simulink model "MotionControl"  (R2014a)
settings: Solver=ode45  StartTime=0.0  StopTime=40  FixedStep=0.00001  RelTol=1e-3
settings Model: Creator=faezeh  LastModifiedBy=faezeh

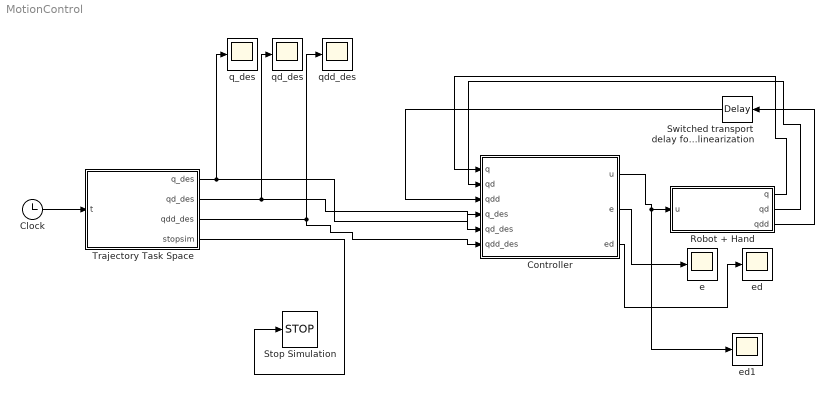
== system MotionControl ==
  Clock : Clock
  Controller : MATLAB Function  TreatAsAtomicUnit=on
  "Robot + Hand " : Subsystem
  Stop Simulation : Stop
  Switched transport delay for linearization : TransportDelay  DelayTime=0.001  TransDelayFeedthrough=on  PadeOrder=2
  Trajectory Task Space : MATLAB Function  TreatAsAtomicUnit=on
  e : Scope
      settings: YMin=-0.0025  YMax=0.0525  SaveName=ScopeData3
  ed : Scope
      settings: TimeRange=40  YMin=-0.05  YMax=1.1  SaveName=ScopeData4
  ed1 : Scope
      settings: YMin=0.00025  YMax=0.00425  SaveName=ScopeData5
  q_des : Scope
      settings: YMin=0.00025  YMax=0.00425
  qd_des : Scope
  qdd_des : Scope
      settings: SaveName=ScopeData2
  wires:
  Clock/1 -> Trajectory Task Space/1(t)
  Trajectory Task Space/1(q_des) -> q_des/1, Controller/4(q_des)
  Trajectory Task Space/2(qd_des) -> qd_des/1, Controller/5(qd_des)
  Trajectory Task Space/3(qdd_des) -> qdd_des/1, Controller/6(qdd_des)
  Controller/1(u) -> ed1/1, "Robot + Hand "/1("u ")
  Trajectory Task Space/4(stopsim) -> Stop Simulation/1
  "Robot + Hand "/1(q) -> Controller/1(q)
  "Robot + Hand "/2(qd) -> Controller/2(qd)
  Controller/2(e) -> e/1
  Controller/3(ed) -> ed/1
  "Robot + Hand "/3(qdd) -> Switched transport delay for linearization/1
  Switched transport delay for linearization/1 -> Controller/3(qdd)

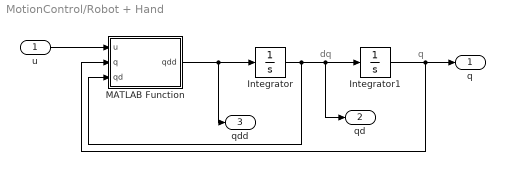
== system MotionControl/Robot + Hand  ==
  note: q
  note: dq
  "u " : Inport
  Integrator : Integrator  InitialCondition=[0.0;0.0;0.0]
  Integrator1 : Integrator  InitialCondition=[0.0;0.0;0.0]
  MATLAB Function : MATLAB Function  TreatAsAtomicUnit=on
  q : Outport
  qd : Outport  Port=2
  qdd : Outport  Port=3
  wires:
  "u "/1 -> MATLAB Function/1(u)
  Integrator/1 -> MATLAB Function/3(qd), qd/1, Integrator1/1
  Integrator1/1 -> MATLAB Function/2(q), q/1
  MATLAB Function/1(qdd) -> qdd/1, Integrator/1

== matlab function MotionControl/Robot + Hand /MATLAB Function ==
  data: u input; qdd output; q input; qd input
function qdd = DirDyn(u,q,qd)
%% Recalling Model Dynamics 
[M,V,G] = DynamicModel(q,qd);
B=[0.0252; 0.0019; 0.0029]; %Nms/rad
Fk=[0.1891; 0.0541; 0.1339]*0;
Jmeta=35.9*0.9*0.9*[1;1;1]*0.001*0.0001;
M=M+[Jmeta(1) 0 0;0 Jmeta(2) 0;0 0 Jmeta(3)]; 
%% Recalling Model Dynamics 
% [~,J,~] = DH2TF(q(1),q(2),q(3));
q1=q(1); q2=q(2); q3=q(3);
J=[ 0,        0,                       0
 0,        0,                       0
 0,        0,                       0
 0, -sin(q1), -cos(q1)*sin(q2 - pi/2)
 0,  cos(q1), -sin(q1)*sin(q2 - pi/2)
 1,        0,          cos(q2 - pi/2)];
fg = -4.98 + 16.92./((1+q./8.59).^2.24);
tawe = fg*66.457*0.001;
qdd =inv(M)*(u -(V + G + B.*qd + Fk.*sign(qd) + tawe));

== matlab function MotionControl/Controller ==
  data: q input; u output; qd input; qdd input; q_des input; qd_des input; qdd_des input; e output; ed output
function [u,e,ed] =Commanand (q,qd,qdd,q_des,qd_des,qdd_des)
    %% Recalling Model Dynamics 
    [M,V,G] = DynamicModel(q,qd);
    B=[0.0252; 0.0019; 0.0029]; %Nms/rad
    Fk=[0.1891; 0.0541; 0.1339]*0; %Nm
    Jmeta=35.9*0.9*0.9*[1;1;1]*0.001*0.0001;
    M=M+[Jmeta(1) 0 0;0 Jmeta(2) 0;0 0 Jmeta(3)];
%     qdd=[0;0;0];
    %% Recalling Model Kinematics
%     [~,J,~] = DH2TF(q(1),q(2),q(3));
    q1=q(1); q2=q(2); q3=q(3);
%     J=[ 0,        0,                    0
%      0,        0,                       0
%      0,        0,                       0
%      0, -sin(q1), -cos(q1)*sin(q2 - pi/2)
%      0,  cos(q1), -sin(q1)*sin(q2 - pi/2)
%      1,        0,          cos(q2 - pi/2)];
    %% Controller Command
    kp=4000;
    kd=1000;
%     q=[0;0;0];
%     qd=[0;0;0];   
u = M*(qdd_des+kd*(qd_des-qd)+kp*(q_des-q)) + V + G + B.*qd + Fk.*sign(qd);  
e=q_des-q;
    ed=qd_des-qd;

== matlab function MotionControl/Trajectory Task Space ==
  data: t input; q_des output; qd_des output; qdd_des output; stopsim output
function [q_des,qd_des,qdd_des,stopsim] = TRJ(t)
   %% trapezoidal velocity profile 
   qf=[50;70;60];
   qf=qf*(pi/180);
   qi=[0;0;0];
   qi=qi*(pi/180);
   L=norm(qf-qi);
   qd_max=0.2; %v_max enterd by user
   T=10;
   qdd_max=qd_max^2/(T*qd_max-L);
   sig=0;
   sigd=0;
   sigdd=0;
   stopsim=0;

   Ts=qd_max/qdd_max;
   if t<=Ts
   sig=qdd_max*t^2/2;
   sigd=qdd_max*t;
   sigdd=qdd_max;
   elseif t>Ts && t<=(T-Ts)
   sig=qd_max*t-(qd_max)^2/(2*qdd_max);
   sigd=qd_max;
   sigdd=0;
   elseif t>(T-Ts) && t<=T
   sig=-qdd_max*(t-T)^2/2+qd_max*T-(qd_max)^2/qdd_max;
   sigd=-qdd_max*(t-T);
   sigdd=-qdd_max;
   else 
    stopsim=1;
   end

   %% Line Trajecory 
   q_des = qi + sig*(qf-qi)/L;
   qd_des = (qf-qi)*sigd/L;
   qdd_des = (qf-qi)*sigdd/L;
end
